simulink model "calcola_A1"  (R2017a)
settings: Solver=FixedStepAuto  StartTime=0.0  StopTime=inf  FixedStep=Tc  RelTol=1e-3
values from neighbouring files (symbols this model uses):
  K = Y(end)    [metodo_aree.m]    (also in stima_grafica_I_ordine.m)
libraries: simulink x2, cstblocks x1
settings Model: Creator=Enrico Donato  LastModifiedBy=Enrico Donato

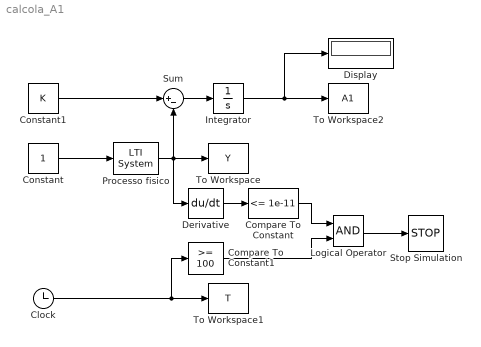
== system calcola_A1 ==
  Clock : Clock
  Compare To Constant : simulink/Logic and Bit Operations/Compare To Constant  relop=<=  const=1e-11  OutDataTypeStr=boolean
  Compare To Constant1 : simulink/Logic and Bit Operations/Compare To Constant  relop=>=  const=100  OutDataTypeStr=boolean
  Constant : Constant
  Constant1 : Constant  Value=K
  Derivative : Derivative
  Display : Display
  Integrator : Integrator
  Logical Operator : Logic  AllPortsSameDT=off  OutDataTypeStr=boolean
  Processo fisico : cstblocks/LTI System  sys=G  IC=[]
  Stop Simulation : Stop
  Sum : Sum  Inputs=|+-
  To Workspace : ToWorkspace  VariableName=Y  SampleTime=-1
  To Workspace1 : ToWorkspace  VariableName=T  SampleTime=-1
  To Workspace2 : ToWorkspace  VariableName=A1  SampleTime=-1
  wires:
  Constant/1 -> Processo fisico/1
  Processo fisico/1 -> Derivative/1, Sum/2, To Workspace/1
  Clock/1 -> To Workspace1/1, Compare To Constant1/1
  Derivative/1 -> Compare To Constant/1
  Compare To Constant/1 -> Logical Operator/1
  Logical Operator/1 -> Stop Simulation/1
  Compare To Constant1/1 -> Logical Operator/2
  Constant1/1 -> Sum/1
  Sum/1 -> Integrator/1
  Integrator/1 -> Display/1, To Workspace2/1
